simulink model "RLC_SIM"  (R2020b)
settings: Solver=VariableStepAuto  StartTime=0.0  StopTime=10.0  RelTol=1e-3
values from neighbouring files (symbols this model uses):
  C = 1    [RLCScript.m]
  L = 1    [RLCScript.m]
  R = 2    [RLCScript.m]
  v = 5    [RLCScript.m]
settings Model: Creator=Arturo Chavez  LastModifiedBy=Arturo Chavez

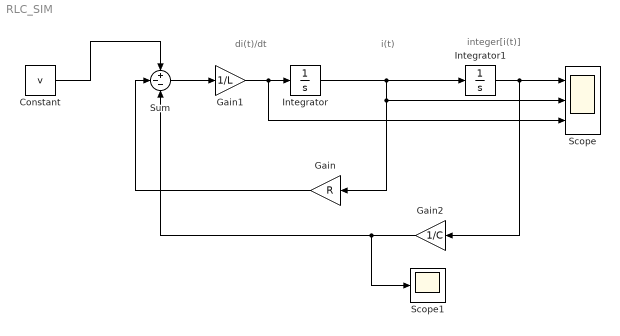
== system RLC_SIM ==
  note: i(t)
  note: di(t)/dt
  note: integer[i(t)]
  Constant : Constant  Value=v
  Gain : Gain  Gain=R
  Gain1 : Gain  Gain=1/L
  Gain2 : Gain  Gain=1/C
  Integrator : Integrator
  Integrator1 : Integrator
  Scope : Scope  NumInputPorts=3
  Scope1 : Scope
  Sum : Sum  Inputs=+--
  wires:
  Constant/1 -> Sum/1
  Integrator/1 -> Scope/2, Gain/1, Integrator1/1
  Integrator1/1 -> Scope/1, Gain2/1
  Gain/1 -> Sum/2
  Gain2/1 -> Scope1/1, Sum/3
  Sum/1 -> Gain1/1
  Gain1/1 -> Scope/3, Integrator/1
